simulink library "mvt_blocks"  (Simulink 3.00)
values from neighbouring files (symbols this model uses):
  stack = struct('general',[],'evaluation',[],'simulation',[],'temp',[])    [gohome.m]
libraries: mvt_blocks x1
(part 2 of 2)

== system mvt_blocks/out7 ==
  Y : Inport  Port=1  PortWidth=-1  SampleTime=0  DataType=auto
      settings: SignalType=auto
  YR : Inport  Port=2  PortWidth=-1  SampleTime=0  DataType=auto
      settings: SignalType=auto
   {1..7} (7 alike) : Scope
      " 1" settings: Orientation=up  TimeRange=100.000000  YMin=-2  YMax=2  SaveToWorkspace=off  SaveName=ScopeData  DataFormat=Matrix
      " 2" settings: Orientation=up  TimeRange=100.000000  YMin=-2.000000  YMax=2.000000  SaveToWorkspace=off  SaveName=ScopeData  DataFormat=Matrix
      " 3" settings: Orientation=up  TimeRange=100.000000  YMin=-2.000000  YMax=2.000000  SaveToWorkspace=off  SaveName=ScopeData  DataFormat=Matrix
      " 4" settings: Orientation=up  TimeRange=100.000000  YMin=-2.000000  YMax=2.000000  SaveToWorkspace=off  SaveName=ScopeData  DataFormat=Matrix
      " 5" settings: Orientation=up  TimeRange=100.000000  YMin=-2.000000  YMax=2.000000  SaveToWorkspace=off  SaveName=ScopeData  DataFormat=Matrix
      " 6" settings: Orientation=up  TimeRange=100.000000  YMin=-2.000000  YMax=2.000000  SaveToWorkspace=off  SaveName=ScopeData  DataFormat=Matrix
      " 7" settings: Orientation=up  TimeRange=100.000000  YMin=-2.000000  YMax=2.000000  SaveToWorkspace=off  SaveName=ScopeData  DataFormat=Matrix
  Demux : Demux  Outputs=7
  Demux1 : Demux  Outputs=7
  Mux{,1..6} (7 alike) : Mux  Orientation=up  Inputs=2
  wires:
  Y/1 -> Demux/1
  Mux/1 -> " 1"/1
  Mux1/1 -> " 2"/1
  Mux2/1 -> " 3"/1
  Demux/3 -> Mux2/1
  Demux/1 -> Mux/1
  YR/1 -> Demux1/1
  Demux1/2 -> Mux1/2
  Demux1/3 -> Mux2/2
  Mux3/1 -> " 4"/1
  Demux1/4 -> Mux3/2
  Demux/2 -> Mux1/1
  Demux/5 -> Mux4/1
  Demux1/5 -> Mux4/2
  Mux4/1 -> " 5"/1
  Mux5/1 -> " 6"/1
  Demux/6 -> Mux5/1
  Demux1/6 -> Mux5/2
  Demux1/1 -> Mux/2
  Mux6/1 -> " 7"/1
  Demux/7 -> Mux6/1
  Demux1/7 -> Mux6/2
  Demux/4 -> Mux3/1

== system mvt_blocks/out8 ==
  Y : Inport  Port=1  PortWidth=-1  SampleTime=0  DataType=auto
      settings: SignalType=auto
  YR : Inport  Port=2  PortWidth=-1  SampleTime=0  DataType=auto
      settings: SignalType=auto
   {1..8} (8 alike) : Scope
      " 1" settings: Orientation=up  TimeRange=100.000000  YMin=-2  YMax=2  SaveToWorkspace=off  SaveName=ScopeData  DataFormat=Matrix
      " 2" settings: Orientation=up  TimeRange=100.000000  YMin=-2.000000  YMax=2.000000  SaveToWorkspace=off  SaveName=ScopeData  DataFormat=Matrix
      " 3" settings: Orientation=up  TimeRange=100.000000  YMin=-2.000000  YMax=2.000000  SaveToWorkspace=off  SaveName=ScopeData  DataFormat=Matrix
      " 4" settings: Orientation=up  TimeRange=100.000000  YMin=-2.000000  YMax=2.000000  SaveToWorkspace=off  SaveName=ScopeData  DataFormat=Matrix
      " 5" settings: Orientation=up  TimeRange=100.000000  YMin=-2.000000  YMax=2.000000  SaveToWorkspace=off  SaveName=ScopeData  DataFormat=Matrix
      " 6" settings: Orientation=up  TimeRange=100.000000  YMin=-2.000000  YMax=2.000000  SaveToWorkspace=off  SaveName=ScopeData  DataFormat=Matrix
      " 7" settings: Orientation=up  TimeRange=100.000000  YMin=-2.000000  YMax=2.000000  SaveToWorkspace=off  SaveName=ScopeData  DataFormat=Matrix
      " 8" settings: Orientation=up  TimeRange=100.000000  YMin=-2.000000  YMax=2.000000  SaveToWorkspace=off  SaveName=ScopeData  DataFormat=Matrix
  Demux : Demux  Outputs=8
  Demux1 : Demux  Outputs=8
  Mux{,1..7} (8 alike) : Mux  Orientation=up  Inputs=2
  wires:
  Y/1 -> Demux/1
  Mux/1 -> " 1"/1
  Demux/3 -> Mux2/1
  YR/1 -> Demux1/1
  Demux1/2 -> Mux1/2
  Demux1/3 -> Mux2/2
  Demux/4 -> Mux3/1
  Demux1/4 -> Mux3/2
  Demux/2 -> Mux1/1
  Demux/5 -> Mux4/1
  Demux1/5 -> Mux4/2
  Demux/6 -> Mux5/1
  Demux1/6 -> Mux5/2
  Demux1/1 -> Mux/2
  Demux/7 -> Mux6/1
  Demux1/7 -> Mux6/2
  Mux1/1 -> " 2"/1
  Mux3/1 -> " 4"/1
  Mux4/1 -> " 5"/1
  Mux5/1 -> " 6"/1
  Mux6/1 -> " 7"/1
  Mux7/1 -> " 8"/1
  Demux/8 -> Mux7/1
  Demux1/8 -> Mux7/2
  Demux/1 -> Mux/1
  Mux2/1 -> " 3"/1

== system mvt_blocks/out9 ==
  Y : Inport  Port=1  PortWidth=-1  SampleTime=0  DataType=auto
      settings: SignalType=auto
  YR : Inport  Port=2  PortWidth=-1  SampleTime=0  DataType=auto
      settings: SignalType=auto
   {1..9} (9 alike) : Scope
      " 1" settings: Orientation=up  TimeRange=100.000000  YMin=-2  YMax=2  SaveToWorkspace=off  SaveName=ScopeData  DataFormat=Matrix
      " 2" settings: Orientation=up  TimeRange=100.000000  YMin=-2.000000  YMax=2.000000  SaveToWorkspace=off  SaveName=ScopeData  DataFormat=Matrix
      " 3" settings: Orientation=up  TimeRange=100.000000  YMin=-2.000000  YMax=2.000000  SaveToWorkspace=off  SaveName=ScopeData  DataFormat=Matrix
      " 4" settings: Orientation=up  TimeRange=100.000000  YMin=-2.000000  YMax=2.000000  SaveToWorkspace=off  SaveName=ScopeData  DataFormat=Matrix
      " 5" settings: Orientation=up  TimeRange=100.000000  YMin=-2.000000  YMax=2.000000  SaveToWorkspace=off  SaveName=ScopeData  DataFormat=Matrix
      " 6" settings: Orientation=up  TimeRange=100.000000  YMin=-2.000000  YMax=2.000000  SaveToWorkspace=off  SaveName=ScopeData  DataFormat=Matrix
      " 7" settings: Orientation=up  TimeRange=100.000000  YMin=-2.000000  YMax=2.000000  SaveToWorkspace=off  SaveName=ScopeData  DataFormat=Matrix
      " 8" settings: Orientation=up  TimeRange=100.000000  YMin=-2.000000  YMax=2.000000  SaveToWorkspace=off  SaveName=ScopeData  DataFormat=Matrix
      " 9" settings: Orientation=up  TimeRange=100.000000  YMin=-2.000000  YMax=2.000000  SaveToWorkspace=off  SaveName=ScopeData  DataFormat=Matrix
  Demux : Demux  Outputs=9
  Demux1 : Demux  Outputs=9
  Mux{,1..8} (9 alike) : Mux  Orientation=up  Inputs=2
  wires:
  Y/1 -> Demux/1
  Mux/1 -> " 1"/1
  Demux/3 -> Mux2/1
  YR/1 -> Demux1/1
  Demux1/2 -> Mux1/2
  Demux1/3 -> Mux2/2
  Demux/4 -> Mux3/1
  Demux1/4 -> Mux3/2
  Demux/2 -> Mux1/1
  Demux/5 -> Mux4/1
  Demux1/5 -> Mux4/2
  Demux/6 -> Mux5/1
  Demux1/6 -> Mux5/2
  Demux/7 -> Mux6/1
  Demux1/7 -> Mux6/2
  Mux1/1 -> " 2"/1
  Mux2/1 -> " 3"/1
  Mux3/1 -> " 4"/1
  Mux4/1 -> " 5"/1
  Mux5/1 -> " 6"/1
  Mux6/1 -> " 7"/1
  Mux7/1 -> " 8"/1
  Demux/8 -> Mux7/1
  Demux1/8 -> Mux7/2
  Demux1/1 -> Mux/2
  Mux8/1 -> " 9"/1
  Demux/9 -> Mux8/1
  Demux1/9 -> Mux8/2
  Demux/1 -> Mux/1

== system mvt_blocks/quasistatic_sp ==
  note: dX2/dt
  note: U
  note: X1
  note: QUASI-STATIC SET POINT COMPUTATION
  Y* : Inport  Port=1  PortWidth=-1  SampleTime=0  DataType=auto
      settings: SignalType=auto
  Matrix Gain2 : Subsystem  mask(Matrix Gain){K=stack.simulation.A21}
      mask prompts: K "Gain matrix:"
      mask help: Matrix Gain.
      mask Help: Multiplies input vector by entered matrix to produce output vector (y=Au).
      mask Display: disp('A21')
  Matrix Gain3 : Subsystem  mask(Matrix Gain){K=stack.simulation.B2}
      mask prompts: K "Gain matrix:"
      mask help: Matrix Gain.
      mask Help: Multiplies input vector by entered matrix to produce output vector (y=Au).
      mask Display: disp('B2')
  Matrix Gain4 : Subsystem  Orientation=left  mask(Matrix Gain){K=stack.simulation.S11*stack.simulation.A12}
      mask prompts: K "Gain matrix:"
      mask help: Matrix Gain.
      mask Help: Multiplies input vector by entered matrix to produce output vector (y=Au).
      mask Display: disp('S11 * A12')
  Matrix Gain5 : Subsystem  Orientation=left  mask(Matrix Gain){K=stack.simulation.S21*stack.simulation.A12}
      mask prompts: K "Gain matrix:"
      mask help: Matrix Gain.
      mask Help: Multiplies input vector by entered matrix to produce output vector (y=Au).
      mask Display: disp('S21 * A12')
  State-Space : Subsystem
      mask Display: disp('I / s')
  Subsystem : Subsystem
      mask Display: disp('[ S12 ]\n[ S22 ]')
  Subsystem1 : Subsystem
      mask Display: disp('inv(T)')
  Sum : Sum  Inputs=-+  SaturateOnIntegerOverflow=on
  Sum1 : Sum  Inputs=+-  SaturateOnIntegerOverflow=on
  Sum2 : Sum  Inputs=++  SaturateOnIntegerOverflow=on
  X* : Outport  Port=1
  U* : Outport  Port=2
  wires:
  Sum1/1 -> U*/1, Matrix Gain3/1(In1)
  Y*/1 -> Subsystem/1(Y*)
  Subsystem1/1(X*) -> X*/1
  Subsystem/1(out_1) -> Sum/2
  Subsystem/2(out_2) -> Sum1/1
  Matrix Gain2/1(Out1) -> Sum2/1
  Matrix Gain3/1(Out1) -> Sum2/2
  Sum2/1 -> State-Space/1(In1)
  Matrix Gain4/1(Out1) -> Sum/1
  Matrix Gain5/1(Out1) -> Sum1/2
  State-Space/1(Out1) -> Matrix Gain4/1(In1), Matrix Gain5/1(In1), Subsystem1/2(X2)
  Sum/1 -> Subsystem1/1(X1), Matrix Gain2/1(In1)

== system mvt_blocks/sf_setpoint ==
  note: X*
  note: U*
  In1 : Inport  Orientation=left  Port=1  PortWidth=-1  SampleTime=-1  DataType=auto
      settings: SignalType=auto
  Matrix Gain : Subsystem  Orientation=left  mask(Matrix Gain){K=stack.simulation.Ksf}
      mask prompts: K "Gain matrix:"
      mask help: Matrix Gain.
      mask Help: Multiplies input vector by entered matrix to produce output vector (y=Au).
      mask Display: disp('Kfb')
  Sum : Sum  Orientation=left  Inputs=|++  SaturateOnIntegerOverflow=on
  setpoint : Subsystem  Orientation=left
      mask Display: disp('SET POINT')
  Out1 : Outport  Orientation=left  Port=1
  wires:
  Sum/1 -> Out1/1
  setpoint/2(U*) -> Sum/2
  Matrix Gain/1(Out1) -> Sum/1
  setpoint/1(X*) -> Matrix Gain/1(In1)
  In1/1 -> setpoint/1(Y*)

== system mvt_blocks/static_sp ==
  note: STATIC SET POINT COMPUTATION
  Y* : Inport  Orientation=left  Port=1  PortWidth=-1  SampleTime=-1  DataType=auto
      settings: SignalType=auto
  Subsystem : Subsystem  Orientation=left
      mask Display: disp('Omega12\n Omega22')
  X* : Outport  Orientation=left  Port=1
  U* : Outport  Orientation=left  Port=2
  wires:
  Subsystem/1(X*) -> X*/1
  Subsystem/2(U*) -> U*/1
  Y*/1 -> Subsystem/1(Y*)

== system mvt_blocks/emfc_controller/Matrix Gain ==
  In1 : Inport  Port=1  PortWidth=-1  SampleTime=-1  DataType=auto
      settings: SignalType=auto
  State Space : StateSpace  A=[]  B=[]  C=[]  D=K  X0=0
  Out1 : Outport  Port=1
  wires:
  In1/1 -> State Space/1
  State Space/1 -> Out1/1

== system mvt_blocks/emfc_controller/Matrix Gain1 ==
  In1 : Inport  Port=1  PortWidth=-1  SampleTime=-1  DataType=auto
      settings: SignalType=auto
  State Space : StateSpace  A=[]  B=[]  C=[]  D=K  X0=0
  Out1 : Outport  Port=1
  wires:
  In1/1 -> State Space/1
  State Space/1 -> Out1/1

== system mvt_blocks/emfc_kpf/Matrix Gain ==
  In1 : Inport  Port=1  PortWidth=-1  SampleTime=-1  DataType=auto
      settings: SignalType=auto
  State Space : StateSpace  A=[]  B=[]  C=[]  D=K  X0=0
  Out1 : Outport  Port=1
  wires:
  In1/1 -> State Space/1
  State Space/1 -> Out1/1

== system mvt_blocks/emfc_kpf/Matrix Gain1 ==
  In1 : Inport  Port=1  PortWidth=-1  SampleTime=-1  DataType=auto
      settings: SignalType=auto
  State Space : StateSpace  A=[]  B=[]  C=[]  D=K  X0=0
  Out1 : Outport  Port=1
  wires:
  In1/1 -> State Space/1
  State Space/1 -> Out1/1

== system mvt_blocks/emfc_kpf/setpoint ==
  Y* : Inport  Orientation=left  Port=1  PortWidth=-1  SampleTime=0  DataType=auto
      settings: SignalType=auto
  X* : Outport  Orientation=left  Port=1
  U* : Outport  Orientation=left  Port=2

== system mvt_blocks/imfc_kpf/Matrix Gain ==
  In1 : Inport  Port=1  PortWidth=-1  SampleTime=-1  DataType=auto
      settings: SignalType=auto
  State Space : StateSpace  A=[]  B=[]  C=[]  D=K  X0=0
  Out1 : Outport  Port=1
  wires:
  State Space/1 -> Out1/1
  In1/1 -> State Space/1

== system mvt_blocks/imfc_kpf/setpoint ==
  Y* : Inport  Orientation=left  Port=1  PortWidth=-1  SampleTime=0  DataType=auto
      settings: SignalType=auto
  X* : Outport  Orientation=left  Port=1
  U* : Outport  Orientation=left  Port=2

== system mvt_blocks/of_setpoint/SubSystem ==
  X* : Inport  Orientation=left  Port=1  PortWidth=-1  SampleTime=-1  DataType=auto
      settings: SignalType=auto
  U* : Inport  Orientation=left  Port=2  PortWidth=-1  SampleTime=-1  DataType=auto
      settings: SignalType=auto
  Controller : StateSpace  Orientation=left  A=stack.simulation.Ak  B=stack.simulation.Bk  C=stack.simulation.Ck  D=stack.simulation.Dk  X0=0
  Matrix Gain : Subsystem  Orientation=left  mask(Matrix Gain){K=stack.general.C}
      mask prompts: K "Gain matrix:"
      mask help: Matrix Gain.
      mask Help: Multiplies input vector by entered matrix to produce output vector (y=Au).
      mask Display: disp('C')
  Matrix Gain1 : Subsystem  Orientation=left  mask(Matrix Gain){K=stack.general.D}
      mask prompts: K "Gain matrix:"
      mask help: Matrix Gain.
      mask Help: Multiplies input vector by entered matrix to produce output vector (y=Au).
      mask Display: disp('D')
  Sum : Sum  Orientation=left  Inputs=|++  SaturateOnIntegerOverflow=on
  Kof Y* : Outport  Orientation=left  Port=1
  wires:
  X*/1 -> Matrix Gain/1(In1)
  Matrix Gain/1(Out1) -> Sum/1
  Sum/1 -> Controller/1
  Controller/1 -> Kof Y*/1
  U*/1 -> Matrix Gain1/1(In1)
  Matrix Gain1/1(Out1) -> Sum/2

== system mvt_blocks/quasistatic_sp/Matrix Gain2 ==
  In1 : Inport  Port=1  PortWidth=-1  SampleTime=-1  DataType=auto
      settings: SignalType=auto
  State Space : StateSpace  A=[]  B=[]  C=[]  D=K  X0=0
  Out1 : Outport  Port=1
  wires:
  In1/1 -> State Space/1
  State Space/1 -> Out1/1

== system mvt_blocks/quasistatic_sp/Matrix Gain3 ==
  In1 : Inport  Port=1  PortWidth=-1  SampleTime=-1  DataType=auto
      settings: SignalType=auto
  State Space : StateSpace  A=[]  B=[]  C=[]  D=K  X0=0
  Out1 : Outport  Port=1
  wires:
  In1/1 -> State Space/1
  State Space/1 -> Out1/1

== system mvt_blocks/quasistatic_sp/Matrix Gain4 ==
  In1 : Inport  Port=1  PortWidth=-1  SampleTime=-1  DataType=auto
      settings: SignalType=auto
  State Space : StateSpace  A=[]  B=[]  C=[]  D=K  X0=0
  Out1 : Outport  Port=1
  wires:
  In1/1 -> State Space/1
  State Space/1 -> Out1/1

== system mvt_blocks/quasistatic_sp/Matrix Gain5 ==
  In1 : Inport  Port=1  PortWidth=-1  SampleTime=-1  DataType=auto
      settings: SignalType=auto
  State Space : StateSpace  A=[]  B=[]  C=[]  D=K  X0=0
  Out1 : Outport  Port=1
  wires:
  In1/1 -> State Space/1
  State Space/1 -> Out1/1

== system mvt_blocks/quasistatic_sp/State-Space ==
  In1 : Inport  Port=1  PortWidth=-1  SampleTime=-1  DataType=auto
      settings: SignalType=auto
  State-Space : StateSpace  A=zeros(stack.simulation.n_x2,stack.simulation.n_x2)  B=eye(stack.simulation.n_x2,stack.simulation.n_x2)  C=eye(stack.simulation.n_x2,stack.simulation.n_x2)  D=zeros(stack.simulation.n_x2,stack.simulation.n_x2)  X0=0
  Out1 : Outport  Port=1
  wires:
  State-Space/1 -> Out1/1
  In1/1 -> State-Space/1

== system mvt_blocks/quasistatic_sp/Subsystem ==
  Y* : Inport  Port=1  PortWidth=-1  SampleTime=-1  DataType=auto
      settings: SignalType=auto
  Matrix Gain : Subsystem  mask(Matrix Gain){K=stack.simulation.S12}
      mask prompts: K "Gain matrix:"
      mask help: Matrix Gain.
      mask Help: Multiplies input vector by entered matrix to produce output vector (y=Au).
      mask Display: disp('S12')
  Matrix Gain1 : Subsystem  mask(Matrix Gain){K=stack.simulation.S22}
      mask prompts: K "Gain matrix:"
      mask help: Matrix Gain.
      mask Help: Multiplies input vector by entered matrix to produce output vector (y=Au).
      mask Display: disp('S22')
  out_1 : Outport  Port=1
  out_2 : Outport  Port=2
  wires:
  Y*/1 -> Matrix Gain/1(In1), Matrix Gain1/1(In1)
  Matrix Gain1/1(Out1) -> out_2/1
  Matrix Gain/1(Out1) -> out_1/1

== system mvt_blocks/quasistatic_sp/Subsystem1 ==
  X1 : Inport  Port=1  PortWidth=-1  SampleTime=-1  DataType=auto
      settings: SignalType=auto
  X2 : Inport  Port=2  PortWidth=-1  SampleTime=-1  DataType=auto
      settings: SignalType=auto
  Matrix Gain8 : Subsystem  mask(Matrix Gain){K=inv(stack.simulation.T)}
      mask prompts: K "Gain matrix:"
      mask help: Matrix Gain.
      mask Help: Multiplies input vector by entered matrix to produce output vector (y=Au).
      mask Display: disp('inv(T)')
  Mux2 : Mux  Inputs=2
      settings: DisplayOption=none
  X* : Outport  Port=1
  wires:
  X2/1 -> Mux2/2
  Matrix Gain8/1(Out1) -> X*/1
  X1/1 -> Mux2/1
  Mux2/1 -> Matrix Gain8/1(In1)

== system mvt_blocks/sf_setpoint/Matrix Gain ==
  In1 : Inport  Port=1  PortWidth=-1  SampleTime=-1  DataType=auto
      settings: SignalType=auto
  State Space : StateSpace  A=[]  B=[]  C=[]  D=K  X0=0
  Out1 : Outport  Port=1
  wires:
  State Space/1 -> Out1/1
  In1/1 -> State Space/1

== system mvt_blocks/sf_setpoint/setpoint ==
  Y* : Inport  Orientation=left  Port=1  PortWidth=-1  SampleTime=0  DataType=auto
      settings: SignalType=auto
  X* : Outport  Orientation=left  Port=1
  U* : Outport  Orientation=left  Port=2

== system mvt_blocks/static_sp/Subsystem ==
  Y* : Inport  Orientation=left  Port=1  PortWidth=-1  SampleTime=-1  DataType=auto
      settings: SignalType=auto
  Matrix Gain : Subsystem  Orientation=left  mask(Matrix Gain){K=stack.simulation.ome12}
      mask prompts: K "Gain matrix:"
      mask help: Matrix Gain.
      mask Help: Multiplies input vector by entered matrix to produce output vector (y=Au).
      mask Display: disp('omega12')
  Matrix Gain1 : Subsystem  Orientation=left  mask(Matrix Gain){K=stack.simulation.ome22}
      mask prompts: K "Gain matrix:"
      mask help: Matrix Gain.
      mask Help: Multiplies input vector by entered matrix to produce output vector (y=Au).
      mask Display: disp('omega22')
  X* : Outport  Orientation=left  Port=1
  U* : Outport  Orientation=left  Port=2
  wires:
  Matrix Gain/1(Out1) -> X*/1
  Matrix Gain1/1(Out1) -> U*/1
  Y*/1 -> Matrix Gain/1(In1), Matrix Gain1/1(In1)

== system mvt_blocks/of_setpoint/SubSystem/Matrix Gain ==
  In1 : Inport  Port=1  PortWidth=-1  SampleTime=-1  DataType=auto
      settings: SignalType=auto
  State Space : StateSpace  A=[]  B=[]  C=[]  D=K  X0=0
  Out1 : Outport  Port=1
  wires:
  In1/1 -> State Space/1
  State Space/1 -> Out1/1

== system mvt_blocks/of_setpoint/SubSystem/Matrix Gain1 ==
  In1 : Inport  Port=1  PortWidth=-1  SampleTime=-1  DataType=auto
      settings: SignalType=auto
  State Space : StateSpace  A=[]  B=[]  C=[]  D=K  X0=0
  Out1 : Outport  Port=1
  wires:
  In1/1 -> State Space/1
  State Space/1 -> Out1/1

== system mvt_blocks/quasistatic_sp/Subsystem/Matrix Gain ==
  In1 : Inport  Port=1  PortWidth=-1  SampleTime=-1  DataType=auto
      settings: SignalType=auto
  State Space : StateSpace  A=[]  B=[]  C=[]  D=K  X0=0
  Out1 : Outport  Port=1
  wires:
  In1/1 -> State Space/1
  State Space/1 -> Out1/1

== system mvt_blocks/quasistatic_sp/Subsystem/Matrix Gain1 ==
  In1 : Inport  Port=1  PortWidth=-1  SampleTime=-1  DataType=auto
      settings: SignalType=auto
  State Space : StateSpace  A=[]  B=[]  C=[]  D=K  X0=0
  Out1 : Outport  Port=1
  wires:
  In1/1 -> State Space/1
  State Space/1 -> Out1/1

== system mvt_blocks/quasistatic_sp/Subsystem1/Matrix Gain8 ==
  In1 : Inport  Port=1  PortWidth=-1  SampleTime=-1  DataType=auto
      settings: SignalType=auto
  State Space : StateSpace  A=[]  B=[]  C=[]  D=K  X0=0
  Out1 : Outport  Port=1
  wires:
  In1/1 -> State Space/1
  State Space/1 -> Out1/1

== system mvt_blocks/static_sp/Subsystem/Matrix Gain ==
  In1 : Inport  Port=1  PortWidth=-1  SampleTime=-1  DataType=auto
      settings: SignalType=auto
  State Space : StateSpace  A=[]  B=[]  C=[]  D=K  X0=0
  Out1 : Outport  Port=1
  wires:
  In1/1 -> State Space/1
  State Space/1 -> Out1/1

== system mvt_blocks/static_sp/Subsystem/Matrix Gain1 ==
  In1 : Inport  Port=1  PortWidth=-1  SampleTime=-1  DataType=auto
      settings: SignalType=auto
  State Space : StateSpace  A=[]  B=[]  C=[]  D=K  X0=0
  Out1 : Outport  Port=1
  wires:
  In1/1 -> State Space/1
  State Space/1 -> Out1/1
